simulink model "rocky_simulink_model_v2"  (R2022b)
settings: Solver=VariableStepAuto  StartTime=0.0  StopTime=5  RelTol=1e-3
values from neighbouring files (symbols this model uses):
  a = 13.8265132822    [MotorParams.mat]    (also in Rocky_5_closed_loop_poles.m = 13.8265; Rocky_closed_loop_poles_23.m = 13.83; poles_impulse_step.m = 13.83)
  b = 0.0036184905593    [MotorParams.mat]    (also in Rocky_5_closed_loop_poles.m = 0.0036; Rocky_closed_loop_poles_23.m = 0.0036; poles_impulse_step.m = 0.0036)
  g = 9.81    [RockyParams.mat]    (also in Rocky_5_closed_loop_poles.m; Rocky_closed_loop_poles_23.m; poles_impulse_step.m)
  l = 0.436    [RockyParams.mat]    (also in Rocky_5_closed_loop_poles.m; Rocky_closed_loop_poles_23.m; poles_impulse_step.m)
libraries: simulink_extras x4, slpidlib x1
settings Model: Creator=16508  LastModifiedBy=16508
settings SolverCC: AlgebraicLoopSolver=TrustRegion
settings DebuggingCC: UnconnectedInputMsg=warning  UnconnectedOutputMsg=warning  UnconnectedLineMsg=warning  SFMachineParentedDataDiag=warning
settings ModelReferenceCC: EnableRefExpFcnMdlSchedulingChecks=on
settings SFSimCC: CustomCodeUndefinedFunction=UseInterfaceOnly
settings RTWCC: DLArmComputeVersion=19.05

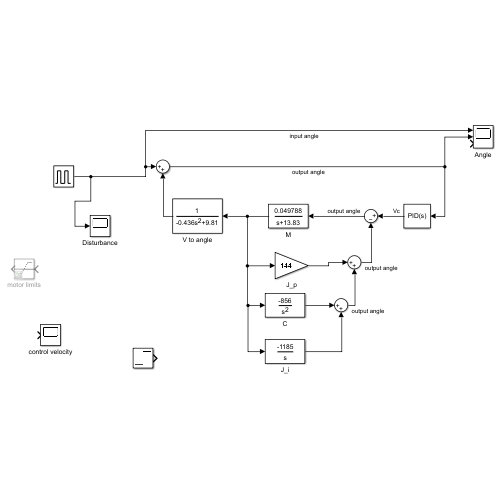
[thumbnail: Simulink's stored preview of the top-level diagram]
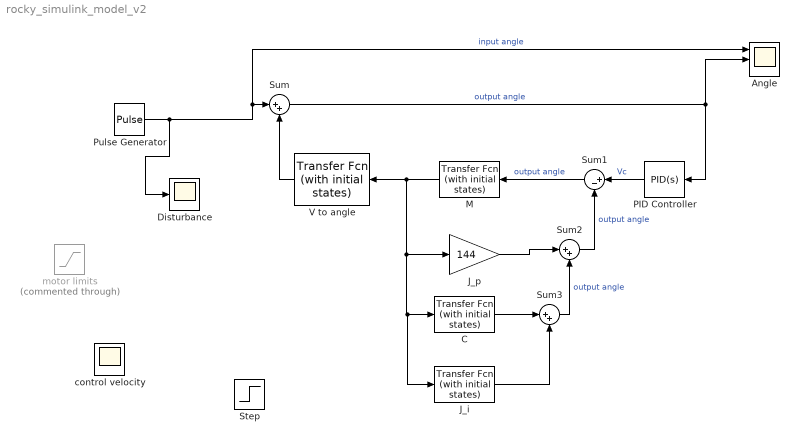
== system rocky_simulink_model_v2 ==
  Angle : Scope  NumInputPorts=3
  C : simulink_extras/Additional Linear/Transfer Fcn (with initial states)  N=[-856]  D=[1 0 0]  X0=0
  Disturbance : Scope
  J_i : simulink_extras/Additional Linear/Transfer Fcn (with initial states)  N=[-1185]  D="[1  0]"  X0=0
  J_p : Gain  Gain=144
  M : simulink_extras/Additional Linear/Transfer Fcn (with initial states)  N=[a*b]  D="[1  a]"  X0=0
  PID Controller : slpidlib/PID Controller  Controller=PID  Form=Parallel  TimeDomain=Continuous-time  UseExternalTs=off  SampleTime=-1  IntegratorMethod=Forward Euler  FilterMethod=Forward Euler  ControllerParametersSource=internal  P=2237  I=10606  UseKiTs=off  D=0  N=100  UseFilter=on  TunerSelectOption=Transfer Function Based (PID Tuner App)  InitialConditionSource=internal  InitialConditionForIntegrator=0  InitialConditionForFilter=0  DifferentiatorICPrevScaledInput=0  ExternalReset=none  TrackingMode=off  Kt=1  LimitOutput=off  SatLimitsSource=internal  UpperSaturationLimit=inf  LowerSaturationLimit=-inf  LinearizeAsGain=on  AntiWindupMode=none  Kb=1  LimitIntegrator=off  UpperIntegratorSaturationLimit=inf  LowerIntegratorSaturationLimit=-inf  POutMin=[]  POutMax=[]  IOutMin=[]  IOutMax=[]  DOutMin=[]  DOutMax=[]  NOutMin=[]  NOutMax=[]  SumOutMin=[]  SumOutMax=[]  SaturationOutMin=[]  SaturationOutMax=[]  PParamMin=[]  PParamMax=[]  IParamMin=[]  IParamMax=[]  DParamMin=[]  DParamMax=[]  NParamMin=[]  NParamMax=[]  KbParamMin=[]  KbParamMax=[]  KtParamMin=[]  KtParamMax=[]  KbOutMin=[]  KbOutMax=[]  KtOutMin=[]  KtOutMax=[]  IntegratorOutMin=[]  IntegratorOutMax=[]  FilterOutMin=[]  FilterOutMax=[]  SumI1OutMin=[]  SumI1OutMax=[]  SumI2OutMin=[]  SumI2OutMax=[]  SumI3OutMin=[]  SumI3OutMax=[]  SumI4OutMin=[]  SumI4OutMax=[]  SumDOutMin=[]  SumDOutMax=[]  DifferentiatorOutMin=[]  DifferentiatorOutMax=[]  FilterDiffOutCoefMin=[]  FilterDiffOutCoefMax=[]  ReciprocalOutMin=[]  ReciprocalOutMax=[]  SumDenOutMin=[]  SumDenOutMax=[]  SumNumOutMin=[]  SumNumOutMax=[]  DivideOutMin=[]  DivideOutMax=[]  UdiffTsProdOutMin=[]  UdiffTsProdOutMax=[]  NTsProdOutMin=[]  NTsProdOutMax=[]  UintegralTsProdOutMin=[]  UintegralTsProdOutMax=[]  UngainTsProdOutMin=[]  UngainTsProdOutMax=[]  ClampingZeroOutDataTypeStr=Inherit: Inherit via back propagation  ClampingZeroOutMin=[]  ClampingZeroOutMax=[]  FilterDenConstantOutDataTypeStr=Inherit: Inherit via back propagation  FilterDenConstantOutMin=[]  FilterDenConstantOutMax=[]  PCopyOutDataTypeStr=Inherit: Inherit via back propagation  PCopyOutMin=[]  PCopyOutMax=[]  NCopyOutDataTypeStr=Inherit: Inherit via back propagation  NCopyOutMin=[]  NCopyOutMax=[]  IntegratorContinuousStateAttributes=''  IntegratorStateMustResolveToSignalObject=off  IntegratorRTWStateStorageClass=Auto  FilterContinuousStateAttributes=''  FilterStateMustResolveToSignalObject=off  FilterRTWStateStorageClass=Auto  ParallelPVariant=InternalParameters  IdealPVariant=Disabled  IVariant=InternalParameters  DVariant=InternalParameters  IntegratorVariant=Continuous  SatVariant=Disabled  AWVariant=Passthrough  PCopyVariant=Disabled  TRVariant=Disabled  FdbkBlocksVariant=Forward  IdealPFdbkVariant=Disabled  SatFdbkVariant=Disabled  DerivativeFilterVariant=ContFilter  NVariant=InternalParameters  NCopyVariant=Disabled  FilterICVariant=InternalICsFilter  IntegratorICVariant=InternalICs  ExternalResetVariant=Disabled  TRSumVariant=Passthrough  SumFdbkVariant=Disabled  SumVariant=Sum_PID  TsampFilterVariant=InternalTs  TsampNgainVariant=Passthrough  TsampIntegralVariant=Passthrough  ExternalSaturationOutDataTypeStr=Inherit: Same as second input
  Pulse Generator : DiscretePulseGenerator  PulseType=Time based  Amplitude=0.1  Period=10  PulseWidth=2  PhaseDelay=1
  Step : Step  After=0.1  SampleTime=0
  Sum : Sum  Inputs=|++
  Sum1 : Sum  Inputs=|+-
  Sum2 : Sum  Inputs=|++
  Sum3 : Sum  Inputs=|++
  V to angle : simulink_extras/Additional Linear/Transfer Fcn (with initial states)  N=[1]  D="[-l 0  g]"  X0=0
  control velocity : Scope
  motor limits : Saturate  Commented=through  UpperLimit=300  LowerLimit=-300
  wires:
  Pulse Generator/1 -> Disturbance/1, Angle/1, Sum/1  "input angle"
  Sum/1 -> Angle/2, PID Controller/1  "output angle"
  PID Controller/1 -> Sum1/1  "Vc"
  M/1 -> J_i/1, C/1, J_p/1, V to angle/1
  V to angle/1 -> Sum/2
  Sum1/1 -> M/1  "output angle"
  J_i/1 -> Sum3/2
  J_p/1 -> Sum2/1
  C/1 -> Sum3/1
  Sum3/1 -> Sum2/2  "output angle"
  Sum2/1 -> Sum1/2  "output angle"
